simulink subsystem "Simulation"  (R2022b)
settings: Solver=VariableStepAuto  StartTime=0.0  StopTime=10.0  RelTol=1e-3
settings Model: Creator=Mario Bertelli  LastModifiedBy=Mario Bertelli

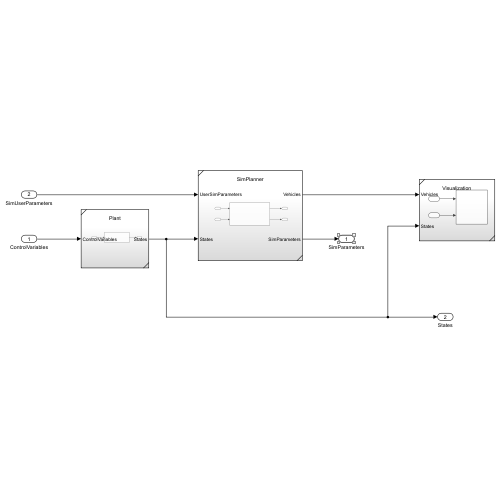
[thumbnail: Simulink's stored preview of the top-level diagram]
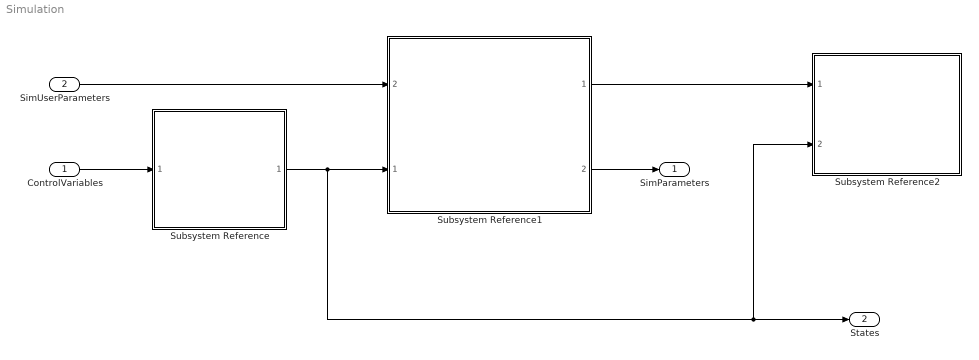
== system Simulation ==
  ControlVariables : Inport
  SimUserParameters : Inport  Port=2
  Subsystem Reference : Subsystem  ReferencedSubsystem=Plant
  Subsystem Reference1 : Subsystem  ReferencedSubsystem=SimPlanner
      settings: PortSchema="{\"entries\":[{\"content\":{\"sides\":[{\"content\":{\"connectorIds\":[\"In2\",\"In1\"]},\"type\":\"ConnectorPlacement.EquallySpacedRectSide\",\"uuid\":\"01c8b9c1-56d7-4050-b5fb-6d9c8034245e\"},{\"content\":{\"connectorIds\":[\"Out1\",\"Out2\"],\"side\":\"RIGHT\"},\"type\":\"ConnectorPlacement.EquallySpacedRectSide\",\"uuid\":\"18ebbf47-1e2e-49a4-8f33-bdc9f37a46af\"},{\"content\":{\"connectorIds\":[],\"side\":\"TOP\"},\"type\":\"ConnectorPlacement.EquallySpacedRectSide\",\"uuid\":\"dccb08d6-820c-420e-b040-0966249e8e89\"}]},\"type\":\"ConnectorPlacement.EquallySpacedConnector\",\"uuid\":\"3cdccb69-d0b7-44c8-a0a2-462917338e25\"}],\"packageUris\":[\"http://schema.mathworks.com/mf0/Connector/R2020b\"],\"version\":\"1.0\"}"
  Subsystem Reference2 : Subsystem  ReferencedSubsystem=Visualization
  SimParameters : Outport
  States : Outport  Port=2
  wires:
  Subsystem Reference/1 -> Subsystem Reference1/1, States/1, Subsystem Reference2/2
  ControlVariables/1 -> Subsystem Reference/1
  Subsystem Reference1/2 -> SimParameters/1
  SimUserParameters/1 -> Subsystem Reference1/2
  Subsystem Reference1/1 -> Subsystem Reference2/1
